simulink model "Centrum_doswiadczalne_2k15"  (R2015a)
settings: Solver=ode3  SolverMode=SingleTasking  StartTime=0.0  StopTime=30.0  FixedStep=0.01  RelTol=1e-3
values from neighbouring files (symbols this model uses):
  p_N_IV = ((z_W'*fi_W)^(-1))*z_W'*yw    [Identyfikacja_parametrow_metoda_bezposrednia_IV_10.m]    (also in Wskazniki_dopasowania_wyswieltenie_danych_11.m = [2.1800, 7.1345, 2.6512, 7.1236])
  p_N_LS = pinv(fi_C)*Z_est_y    [Identyfikacja_parametrow_LS_6.m]    (also in Identyfikacja_parametrow_LS_new_8.m = pinv(fi)*Z_est_y; Identyfikacja_parametrow_metoda_bezposrednia_IV_10.m = [1.9459, 6.9874, 2.4031, 6.9655]; Identyfikacja_parametrow_metoda_bezposrednia_LS_9.m = ((fi_W'*fi_W)^(-1))*fi_W'*yw; Identyfikacja_parametrow_posrednia_LS_delta_plus_6_1.m)
settings Model: CovMetricSettings=dwe  CovHtmlReporting=off  covSaveCumulativeToWorkspaceVar=off  CovSaveSingleToWorkspaceVar=off  CovExternalEMLEnable=on  Creator=mgmil  LastModifiedBy=mgmil
settings DataIOCC: LimitDataPoints=off  SaveFormat=Dataset
settings DebuggingCC: SFUnexpectedBacktrackingDiag=error  SFNoUnconditionalDefaultTransitionDiag=error
settings HardwareCC: ProdBitPerPointer=64  ProdLargestAtomicFloat=Float  ProdIntDivRoundTo=Zero  ProdEndianess=LittleEndian  ProdHWDeviceType=Specified
settings ModelReferenceCC: PropagateSignalLabelsOutOfModel=on
settings SFSimCC: SimUseLocalCustomCode=on
settings RTWCC: RTWUseLocalCustomCode=on
settings GRTTargetCC: TargetLangStandard=C99 (ISO)  GeneratePreprocessorConditionals=Use local settings

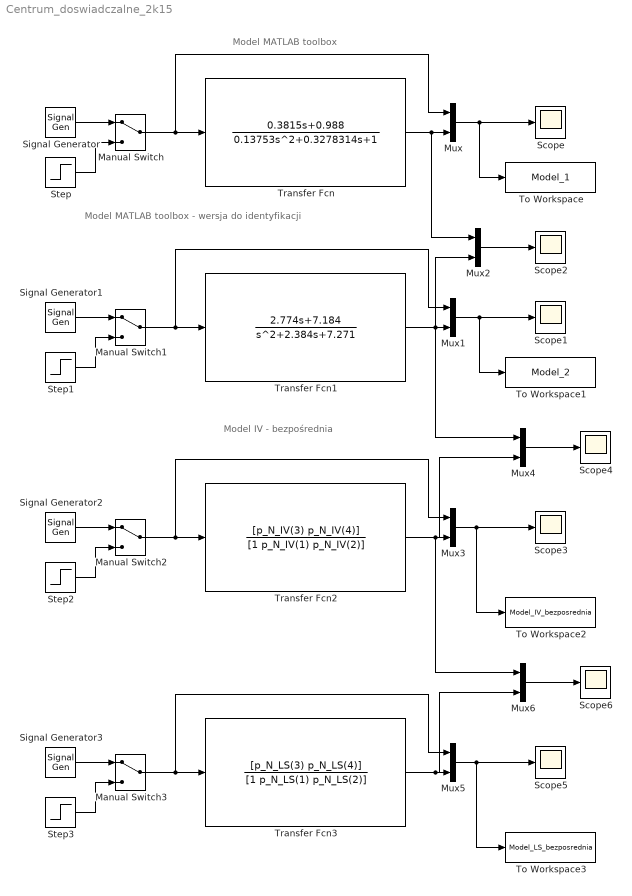
== system Centrum_doswiadczalne_2k15 ==
  note: Model MATLAB toolbox - wersja do identyfikacji
  note: Model MATLAB toolbox
  note: Model IV - bezpośrednia
  Manual Switch{,1..3} (4 alike) : ManualSwitch
  Mux{,1..6} (7 alike) : Mux  Inputs=2
  Scope{,1..6} (7 alike) : Scope
      Scope settings: TimeRange=auto  MaxDataPoints=5000  SaveToWorkspace=off  SaveName=ScopeData  YMin=-2.22676  YMax=3.2967  SampleTime=-1
      Scope1 settings: TimeRange=auto  MaxDataPoints=5000  SaveToWorkspace=off  YMin=-2.22676  YMax=3.2967  SampleTime=-1
      Scope2 settings: TimeRange=auto  MaxDataPoints=5000  SaveToWorkspace=off  SaveName=ScopeData2  YMin=-2.22676  YMax=3.2967  SampleTime=-1
      Scope3 settings: TimeRange=auto  MaxDataPoints=5000  SaveToWorkspace=off  YMin=-2.22676  YMax=3.2967  SampleTime=-1
      Scope4 settings: TimeRange=auto  MaxDataPoints=5000  SaveToWorkspace=off  SaveName=ScopeData2  YMin=1.52725  YMax=2.06552  SampleTime=-1
      Scope5 settings: TimeRange=auto  MaxDataPoints=5000  SaveToWorkspace=off  YMin=-2.22676  YMax=3.2967  SampleTime=-1
      Scope6 settings: TimeRange=auto  MaxDataPoints=5000  SaveToWorkspace=off  SaveName=ScopeData2  YMin=-2.34724  YMax=2.35013  SampleTime=-1
  Signal Generator{,1..3} (4 alike) : SignalGenerator  WaveForm=square  Frequency=0.1
  Step{,1..3} (4 alike) : Step  Time=0  Before=-1  SampleTime=0
  To Workspace : ToWorkspace  VariableName=Model_1  SampleTime=-1
  To Workspace1 : ToWorkspace  VariableName=Model_2  SampleTime=-1
  To Workspace2 : ToWorkspace  VariableName=Model_IV_bezposrednia  SampleTime=-1
  To Workspace3 : ToWorkspace  VariableName=Model_LS_bezposrednia  SampleTime=-1
  Transfer Fcn : TransferFcn  Numerator=[0.3815 0.988]  Denominator=[0.13753 0.3278314 1]
  Transfer Fcn1 : TransferFcn  Numerator=[2.774 7.184]  Denominator=[1 2.384 7.271]
  Transfer Fcn2 : TransferFcn  Numerator=[p_N_IV(3) p_N_IV(4)]  Denominator=[1 p_N_IV(1) p_N_IV(2)]
  Transfer Fcn3 : TransferFcn  Numerator=[p_N_LS(3) p_N_LS(4)]  Denominator=[1 p_N_LS(1) p_N_LS(2)]
  wires:
  Transfer Fcn/1 -> Mux2/1, Mux/2
  Signal Generator/1 -> Manual Switch/1
  Mux/1 -> To Workspace/1, Scope/1
  Manual Switch/1 -> Mux/1, Transfer Fcn/1
  Step/1 -> Manual Switch/2
  Step1/1 -> Manual Switch1/2
  Manual Switch1/1 -> Mux1/1, Transfer Fcn1/1
  Signal Generator1/1 -> Manual Switch1/1
  Mux1/1 -> To Workspace1/1, Scope1/1
  Mux2/1 -> Scope2/1
  Signal Generator2/1 -> Manual Switch2/1
  Mux3/1 -> To Workspace2/1, Scope3/1
  Manual Switch2/1 -> Mux3/1, Transfer Fcn2/1
  Step2/1 -> Manual Switch2/2
  Transfer Fcn2/1 -> Mux6/1, Mux4/2, Mux3/2
  Mux4/1 -> Scope4/1
  Transfer Fcn1/1 -> Mux4/1, Mux2/2, Mux1/2
  Signal Generator3/1 -> Manual Switch3/1
  Manual Switch3/1 -> Mux5/1, Transfer Fcn3/1
  Transfer Fcn3/1 -> Mux6/2, Mux5/2
  Mux5/1 -> To Workspace3/1, Scope5/1
  Step3/1 -> Manual Switch3/2
  Mux6/1 -> Scope6/1
